simulink model "MSE312_Lab4_Ex4_1"  (R2023a)
settings: Solver=ode5  StartTime=0.0  StopTime=inf  FixedStep=0.01  RelTol=1e-3  EnableMultiTasking=on
libraries: arduinolib x2, SignalEditorBlockLib x1, simulink x1, arduinosensorlib x1, eeGeneralControl x1, RASPlib x1
settings Model: ExtModeTrigDuration=2  Creator=mwa140  LastModifiedBy=mwa140
settings OptimizationCC: EnhancedBackFolding=on  PassReuseOutputArgsAs=Individual arguments  ZeroExternalMemoryAtStartup=off  ZeroInternalMemoryAtStartup=off  MaxStackSize=64  OptimizeBlockOrder=speed  DifferentSizesBufferReuse=on  OptimizationCustomize=off  EfficientTunableParamExpr=on
settings DebuggingCC: ParameterTunabilityLossMsg=error
settings HardwareCC: ProdBitPerInt=16  ProdBitPerPointer=16  ProdBitPerSizeT=16  ProdBitPerPtrDiffT=16  ProdLargestAtomicFloat=None  ProdWordSize=8  ProdHWDeviceType=Atmel->AVR
settings SFSimCC: MATLABDynamicMemAlloc=off
settings RTWCC: Description=Embedded Coder  SystemTargetFile=ert.tlc  HardwareBoard=Arduino Mega 2560  TemplateMakefile=ert_default_tmf  Toolchain=Arduino AVR  BuildConfiguration=Faster Runs
settings CodeAppCC: ForceParamTrailComments=on  IgnoreCustomStorageClasses=off  OperatorAnnotations=on  SimulinkDataObjDesc=on  SFDataObjDesc=on  InsertBlockDesc=on
settings ERTTargetCC: SupportContinuousTime=on  SupportVariableSizeSignals=on  ExtModeTransport=3  ExtModeStaticAlloc=on  ExtModeAutomaticAllocSize=off  ExtModeStaticAllocSize=2048  ExtModeMexFile=ext_xcp  ExtModeIntrfLevel=Level2 - Open

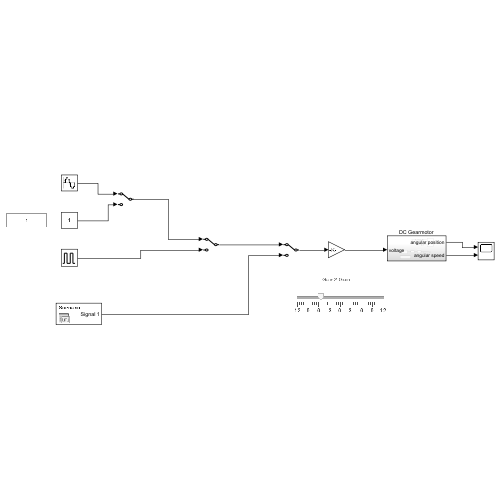
[thumbnail: Simulink's stored preview of the top-level diagram]
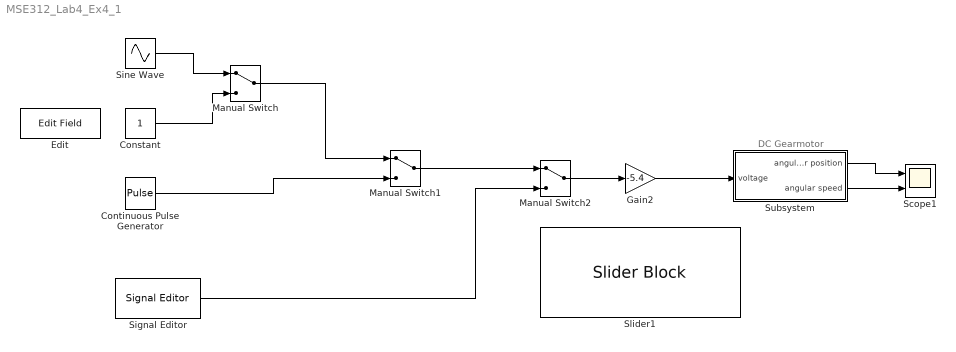
== system MSE312_Lab4_Ex4_1 ==
  note: DC Gearmotor
  Constant : Constant
  Continuous Pulse Generator : DiscretePulseGenerator  PulseType=Time based  PulseWidth=50
  Edit : EditField  LabelPosition=Hide  ShowInitialText=on  Alignment=Center
  Gain2 : Gain  Gain=-5.4
  Manual Switch : ManualSwitch
  Manual Switch1 : ManualSwitch
  Manual Switch2 : ManualSwitch
  Scope1 : Scope  NumInputPorts=2
  Signal Editor : SignalEditorBlockLib/Signal Editor  FileName=MSE312_Lab4_Ex4_1.mat  ActiveScenario=Scenario  ActiveSignal=Signal 1  IsBus=off  OutputBusObjectStr=Bus: BusObject  SampleTime=0  Interpolate=off  ZeroCross=off  OutputAfterFinalValue=Setting to zero  Unit=inherit  PreserveSignalName=on  ApplySigPropsToAllScenarios=on
  Sine Wave : Sin  SampleTime=0.01
  Slider1 : SliderBlock  ScaleMin=-12  ScaleMax=12
  Subsystem : Subsystem
  wires:
  Sine Wave/1 -> Manual Switch/1
  Constant/1 -> Manual Switch/2
  Manual Switch/1 -> Manual Switch1/1
  Manual Switch1/1 -> Manual Switch2/1
  Manual Switch2/1 -> Gain2/1
  Gain2/1 -> Subsystem/1(voltage)
  Continuous Pulse Generator/1 -> Manual Switch1/2
  Signal Editor/1 -> Manual Switch2/2
  Subsystem/2(angular speed) -> Scope1/2
  Subsystem/1(angular position) -> Scope1/1

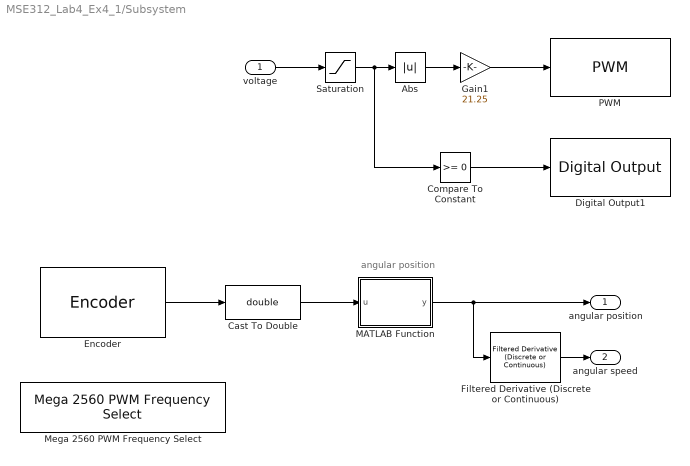
== system MSE312_Lab4_Ex4_1/Subsystem ==
  note: angular position
  voltage : Inport
  Abs : Abs  SaturateOnIntegerOverflow=off
  Cast To Double : DataTypeConversion  OutDataTypeStr=double  SaturateOnIntegerOverflow=off  RndMeth=Floor
  Compare To Constant : simulink/Logic and Bit Operations/Compare To Constant  relop=>=  const=0  OutDataTypeStr=boolean
  Digital Output1 : arduinolib/Digital Output  pinNumber=10  Direction=output  blockPlatform=arduino
  Encoder : arduinosensorlib/Encoder  InputA=2  InputB=3  Mode=No reset  SampleTime=0.01
  Filtered Derivative (Discrete or Continuous) : eeGeneralControl/Filtered Derivative (Discrete or Continuous)  K=1  T=0.1  B=inf  A=-inf  minRatio=10  init_option=Inherited from block input  x0=0  Ts=-1
      settings: LibrarySourceBlock=|
      | ee_sl_lib/General Control/Filtered Derivative
      | (Discrete or Continuous)
  Gain1 : Gain  Gain=21.25
  MATLAB Function : MATLAB Function  TreatAsAtomicUnit=on
  Mega 2560 PWM Frequency Select : RASPlib/Mega 2560 PWM Frequency Select  Frequency=32KHz  Timer=2 - pins 9, 10
      settings: SourceProductName=Rensselaer Arduino Support Package
  PWM : arduinolib/PWM  pinNumber=9  frequencyType=Default  desiredFrequency=490.2  achievableFrequency=490.2
  Saturation : Saturate  UpperLimit=12  LowerLimit=-12
  angular position : Outport
  angular speed : Outport  Port=2
  wires:
  Cast To Double/1 -> MATLAB Function/1(u)
  MATLAB Function/1(y) -> Filtered Derivative (Discrete or Continuous)/1, angular position/1
  Filtered Derivative (Discrete or Continuous)/1 -> angular speed/1
  Saturation/1 -> Compare To Constant/1, Abs/1
  Gain1/1 -> PWM/1
  Abs/1 -> Gain1/1
  Compare To Constant/1 -> Digital Output1/1
  voltage/1 -> Saturation/1
  Encoder/1 -> Cast To Double/1

== matlab function MSE312_Lab4_Ex4_1/Subsystem/MATLAB Function ==
  data: u input; y output
function y = fcn(u)

pos=360/(500*4*6.3);
%pause(1);

y = pos*u;
